simulink model "Seminar6_topic1"  (R2019b)
settings: Solver=ode23tb  StartTime=0.0  StopTime=0.03  MaxStep=1e-5  RelTol=1e-3  AbsTol=.01  EnableMultiTasking=on
libraries: powerlib x15, powerlib_meascontrol x4, simulink x1
settings Model: Creator=ASUS  LastModifiedBy=96547
settings SolverCC: AutoScaleAbsTol=off
settings DataIOCC: LimitDataPoints=on  SaveFormat=Array  SignalLoggingSaveFormat=ModelDataLogs  ReturnWorkspaceOutputs=off
settings OptimizationCC: InitFltsAndDblsToZero=on  LifeSpan=inf
settings DebuggingCC: SaveWithParameterizedLinksMsg=none  UnderspecifiedInitializationDetection=Classic  MergeDetectMultiDrivingBlocksExec=none  SignalResolutionControl=TryResolveAllWithWarning  SolverPrmCheckMsg=warning  MultiTaskDSMMsg=warning  MultiTaskCondExecSysMsg=none  FcnCallInpInsideContextMsg=warning  SFUnexpectedBacktrackingDiag=warning  SFNoUnconditionalDefaultTransitionDiag=warning  ArithmeticOperatorsInVariantConditions=warning
settings HardwareCC: ProdBitPerPointer=32  ProdBitPerSizeT=32  ProdBitPerPtrDiffT=32  ProdLargestAtomicFloat=None  ProdIntDivRoundTo=Undefined  ProdEndianess=Unspecified  ProdWordSize=32  ProdHWDeviceType=32-bit Generic
settings ModelReferenceCC: PropagateSignalLabelsOutOfModel=off
settings SFSimCC: SimUseLocalCustomCode=off  CustomCodeUndefinedFunction=UseInterfaceOnly
settings RTWCC: RTWUseLocalCustomCode=off
settings CodeAppCC: StateflowObjectComments=on
settings GRTTargetCC: TargetFcnLib=ansi_tfl_tmw.mat  TargetLangStandard=C89/C90 (ANSI)  CombineOutputUpdateFcns=off  GRTInterface=on
settings ConfigComp: CovMetricSettings=dw  CovHtmlReporting=on  CovSaveCumulativeToWorkspaceVar=on  CovSaveSingleToWorkspaceVar=on  CovExternalEMLEnable=off
settings SimscapeCC: SimscapeNormalizeSystem=off

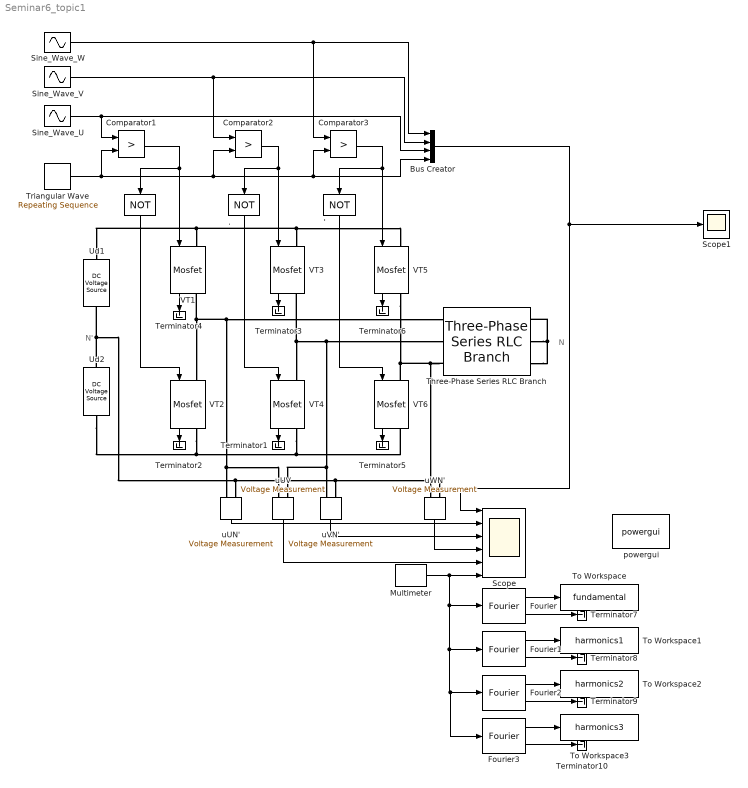
== system Seminar6_topic1 ==
  note: N'
  note: N
  " " : Logic  Operator=NOT  AllPortsSameDT=off  OutDataTypeStr=boolean
  " '" : Logic  Operator=NOT  AllPortsSameDT=off  OutDataTypeStr=boolean
  " ." : Logic  Operator=NOT  AllPortsSameDT=off  OutDataTypeStr=boolean
  Bus Creator : BusCreator  DialogController=Simulink.DDGSource_Bus  Inputs=4
  Comparator1 : RelationalOperator  Operator=>  OutDataTypeStr=boolean  RndMeth=Nearest
  Comparator2 : RelationalOperator  Operator=>  OutDataTypeStr=boolean  RndMeth=Nearest
  Comparator3 : RelationalOperator  Operator=>  OutDataTypeStr=boolean  RndMeth=Nearest
  Fourier : powerlib_meascontrol/Measurements/Fourier  Freq=50  n=1  InInit=[0, 0]  Ts=0
      settings: SourceProductName=Simscape Electrical
  Fourier1 : powerlib_meascontrol/Measurements/Fourier  Freq=6000+2*50  n=1  InInit=[0, 0]  Ts=0
      settings: SourceProductName=Simscape Electrical
  Fourier2 : powerlib_meascontrol/Measurements/Fourier  Freq=2*6000+50  n=1  InInit=[0, 0]  Ts=0
      settings: SourceProductName=Simscape Electrical
  Fourier3 : powerlib_meascontrol/Measurements/Fourier  Freq=3*6000+2*50  n=1  InInit=[0, 0]  Ts=0
      settings: SourceProductName=Simscape Electrical
  Multimeter : powerlib/Measurements/Multimeter  PhasorSimulation=off  OutputType=Complex  sel=1  L=6  Gain=1  yselected={'Ub1: Three-Phase Series RLC Branch'};  PSBOutputType=1  PSBequivalent=0  AxesSetting=[0,0.1,-100,100]  Display=0  SavedBlockNames=-11
      settings: SourceProductName=Simscape Electrical
  Scope : Scope  NumInputPorts=6
  Scope1 : Scope
  Sine_Wave_U : Sin  Amplitude=0.5  Frequency=314  SampleTime=0
  Sine_Wave_V : Sin  Amplitude=0.5  Frequency=314  Phase=-2*pi/3  SampleTime=0
  Sine_Wave_W : Sin  Amplitude=0.5  Frequency=314  Phase=2*pi/3  SampleTime=0
  Terminator{1..10} (10 alike) : Terminator
  Three-Phase Series RLC Branch : powerlib/Elements/Three-Phase Series RLC Branch  LConnTagsString=A|B|C  RConnTagsString=A|B|C  BranchType=RL  Resistance=10  Inductance=0.002  Capacitance=inf  Measurements=Branch voltages and currents
      settings: SourceProductName=Simscape Electrical
  To Workspace : ToWorkspace  VariableName=fundamental  SampleTime=-1
      settings: Save2DSignal=2-D array (concatenate along first dimension)
  To Workspace1 : ToWorkspace  VariableName=harmonics1  SampleTime=-1
      settings: Save2DSignal=2-D array (concatenate along first dimension)
  To Workspace2 : ToWorkspace  VariableName=harmonics2  SampleTime=-1
      settings: Save2DSignal=2-D array (concatenate along first dimension)
  To Workspace3 : ToWorkspace  VariableName=harmonics3  SampleTime=-1
      settings: Save2DSignal=2-D array (concatenate along first dimension)
  Triangular Wave : simulink/Sources/Repeating Sequence  rep_seq_t=[0 0.416e-5 0.833e-4 1.249e-4 1.667e-4]  rep_seq_y=[0 1 0 -1 0]
  Ud1 : powerlib/Electrical Sources/DC Voltage Source  Amplitude=475  Measurements=None
      settings: SourceProductName=Simscape Electrical
  Ud2 : powerlib/Electrical Sources/DC Voltage Source  Amplitude=475  Measurements=None
      settings: SourceProductName=Simscape Electrical
  VT{1..6} (6 alike) : powerlib/Power Electronics/Mosfet  Ron=0.01  Lon=1e-7  Rd=.01  Vfd=0  IC=0  Rs=5  Cs=1e-6  Measurements=on
      settings: SourceProductName=Simscape Electrical
  powergui : powerlib/powergui  Priority=1  SimulationMode=Continuous  SampleTime=50e-6  frequency=60  Iterations=50  frequencyindice=0  Pbase=100e6  ErrMax=1e-4  UnitsV=kV  UnitsW=MW  buscounter=0  FunctionMessages=off  echomessages=off  EnableUseOfTLC=off  CurrentSourceSwitches=on  DisableSnubberDevices=off  DisableRonSwitches=off  DisableVfSwitches=off  DisplayEquations=off  AutomaticDiscreteSolvers=off  SolverType=Tustin/Backward Euler (TBE)  Interpol=off  ExternalGateDelay=off  methode=off  Ts=10  x0status=blocks  SPID=off  SwTol=0  HookPort=off  NonlinearTolerance=1e-4  nMaxIteration=100  ContinueOnMaxIteration=off  RestoreLinks=warning  ResistiveCurrentMeasurement=off  Frange=[0:2:500]  Ylog=off  Xlog=on  ShowGrid=off  save=off  variable=ZData  structure=result_waveform  ZoomFFT=off  StartTime=0.0  cycles=1  DisplayStyle=1  fundamental=50  FreqAxis=off  MaxFrequency=75000  frequencyindicesteady=1  RmsSteady=1  display=off
      settings: SourceProductName=Simscape Electrical
  uUN' : powerlib/Measurements/Voltage Measurement  PhasorSimulation=off  OutputType=Complex  PSBequivalent=0
      settings: SourceProductName=Simscape Electrical
  uUV : powerlib/Measurements/Voltage Measurement  PhasorSimulation=off  OutputType=Complex  PSBequivalent=0
      settings: SourceProductName=Simscape Electrical
  uVN' : powerlib/Measurements/Voltage Measurement  PhasorSimulation=off  OutputType=Complex  PSBequivalent=0
      settings: SourceProductName=Simscape Electrical
  uWN' : powerlib/Measurements/Voltage Measurement  PhasorSimulation=off  OutputType=Complex  PSBequivalent=0
      settings: SourceProductName=Simscape Electrical
  wires:
  Comparator1/1 -> " "/1, VT1/1
  VT4/1 -> Terminator1/1
  VT2/1 -> Terminator2/1
  VT3/1 -> Terminator3/1
  Sine_Wave_U/1 -> Bus Creator/3, Comparator1/1
  Triangular Wave/1 -> Comparator1/2, Comparator2/2, Comparator3/2, Bus Creator/4
  " "/1 -> VT2/1
  Multimeter/1 -> Fourier3/1, Fourier2/1, Fourier1/1, Fourier/1, Scope/6
  VT1/1 -> Terminator4/1
  VT5/1 -> Terminator6/1
  VT6/1 -> Terminator5/1
  Comparator2/1 -> VT3/1, " ."/1
  Comparator3/1 -> VT5/1, " '"/1
  " ."/1 -> VT4/1
  " '"/1 -> VT6/1
  Sine_Wave_V/1 -> Comparator2/1, Bus Creator/2
  Sine_Wave_W/1 -> Comparator3/1, Bus Creator/1
  uUV/1 -> Scope/5
  uWN'/1 -> Scope/4
  uVN'/1 -> Scope/3
  uUN'/1 -> Scope/2
  Bus Creator/1 -> Scope1/1, Scope/1
  Fourier/2 -> Terminator7/1
  Fourier1/2 -> Terminator8/1
  Fourier2/2 -> Terminator9/1
  Fourier3/2 -> Terminator10/1
  Fourier/1 -> To Workspace/1
  Fourier1/1 -> To Workspace1/1
  Fourier2/1 -> To Workspace2/1
  Fourier3/1 -> To Workspace3/1
  connections:
  uUN'/LConn1 -- uUV/LConn1 -- Three-Phase Series RLC Branch/LConn1 -- VT1/RConn1 -- VT2/LConn1
  Ud2/LConn1 -- VT2/RConn1 -- VT6/RConn1 -- VT4/RConn1
  VT3/LConn1 -- VT5/LConn1 -- Ud1/RConn1 -- VT1/LConn1
  Three-Phase Series RLC Branch/LConn3 -- VT6/LConn1 -- VT5/RConn1 -- uWN'/LConn1
  Three-Phase Series RLC Branch/RConn2 -- Three-Phase Series RLC Branch/RConn3 -- Three-Phase Series RLC Branch/RConn1
  Ud2/RConn1 -- Ud1/LConn1 -- uUN'/LConn2 -- uWN'/LConn2 -- uVN'/LConn2
  VT3/RConn1 -- VT4/LConn1 -- Three-Phase Series RLC Branch/LConn2 -- uVN'/LConn1 -- uUV/LConn2
